simulink library "simulink_gym"  (R2020b)
settings: Solver=VariableStepAuto  StartTime=0.0  StopTime=10.0  RelTol=1e-3
undefined symbols (not defined in the file or in its folder): f
libraries: instrumentlib x2
settings Model: Creator=jbrust  LastModifiedBy=jbrust

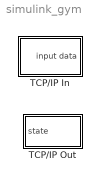
== system simulink_gym ==
  TCP/IP In : Subsystem  mask(TCP/IP In){port=42313, num_signals=2, t_s=1}
      mask prompts: num_signals "Number of input signals:"; t_s "Sample time (-1 for inherited):"
      mask help: TCP/IP block receiving the input and stop signal from the Simulink Gym interface.
  TCP/IP Out : Subsystem  mask(TCP/IP Out){port=42312, t_s=1}
      mask prompts: t_s "Sample time (-1 for inherited):"
      mask help: TCP/IP block sending simulation time and state to the Simulink Gym interface.

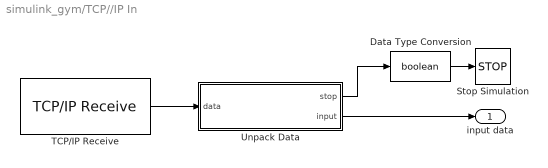
== system simulink_gym/TCP//IP In ==
  Data Type Conversion : DataTypeConversion  OutDataTypeStr=boolean
  Stop Simulation : Stop
  TCP/IP Receive : instrumentlib/TCP//IP Receive  Priority=2  Host=localhost  Port=port  DataSize="[(num_signals + 1)  1]"  EnableBlockingMode=on  Timeout=300  SampleTime=t_s  DataType=double  ByteOrder=LittleEndian  ASCIIFormatting=%f,  Terminator=LF
  Unpack Data : MATLAB Function  Priority=2  TreatAsAtomicUnit=on  SystemSampleTime=t_s
  input data : Outport
  wires:
  Data Type Conversion/1 -> Stop Simulation/1
  TCP/IP Receive/1 -> Unpack Data/1(data)
  Unpack Data/1(stop) -> Data Type Conversion/1
  Unpack Data/2(input) -> input data/1

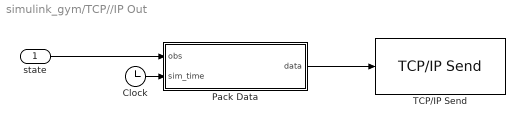
== system simulink_gym/TCP//IP Out ==
  state : Inport
  Clock : Clock
  Pack Data : MATLAB Function  TreatAsAtomicUnit=on  SystemSampleTime=t_s
  TCP/IP Send : instrumentlib/TCP//IP Send  Priority=1  Host=localhost  Port=port  EnableBlockingMode=on  Timeout=300  ByteOrder=LittleEndian  TransferDelay=on
  wires:
  state/1 -> Pack Data/1(obs)
  Clock/1 -> Pack Data/2(sim_time)
  Pack Data/1(data) -> TCP/IP Send/1

== matlab function simulink_gym/TCP//IP In/Unpack Data ==
  data: data input; stop output; input output
function [stop, input] = unpackData(data)
stop = data(1); 
input = data(2:end);

== matlab function simulink_gym/TCP//IP Out/Pack Data ==
  data: obs input; data output; sim_time input
function data = packData(obs, sim_time)
obs = obs(:); % Convert to column vector
data = [double(obs); double(sim_time)];
